simulink model "CF025A_GmFctDiArbn"  (R2013b)
settings: Solver=FixedStepDiscrete  SolverMode=SingleTasking  StartTime=0.0  StopTime=60  FixedStep=0.002  RelTol=1e-3
values from neighbouring files (symbols this model uses):
  GmFctDiArbnEotHwAgThd = DataDict.Calibration    [CF025A_GmFctDiArbn_DataDict.m]
  GmFctDiArbnEotTi = DataDict.Calibration    [CF025A_GmFctDiArbn_DataDict.m]
  GmFctDiArbnOnCentrHwAgThd = DataDict.Calibration    [CF025A_GmFctDiArbn_DataDict.m]
  GmFctDiArbnOnCentrHwTqThd = DataDict.Calibration    [CF025A_GmFctDiArbn_DataDict.m]
  GmFctDiArbnOnCentrTi = DataDict.Calibration    [CF025A_GmFctDiArbn_DataDict.m]
  GmFctDiArbnSrvTi = DataDict.Calibration    [CF025A_GmFctDiArbn_DataDict.m]
  MICROSECTOSEC_ULS_F32 = DataDict.Constant    [CF025A_GmFctDiArbn_DataDict.m]
  ZEROHWAG_HWDEG_F32 = DataDict.Constant    [CF025A_GmFctDiArbn_DataDict.m]
undefined symbols (not defined in the file or in its folder): GmFctDiArbnSts1, LoaSt1
libraries: simulink x7, FixdToFloat x4
(part 2 of 3)

== system CF025A_GmFctDiArbn/GmFctDiArbn/GmFctDiArbnPer1/LoaSt_doesnt_equal_SwBasdMtgtn/ComponentDisable/TimeOut ==
  Action Port : ActionPort  ActionType=then
  Constant{1..5} (5 alike) : Constant  Value=false
  Copyright1 : Subsystem  Description=|  mask(Copyright Information){none=on}
      | Copyright info block.                                               
      |                                                                     
      | Place copyright information at the top of every subsystem in design.
      mask prompts: none "No parameters"
      mask help: Place copyright information at the top of every subsystem in design.
      mask Display:
      | NxtrConf = 'Nexteer Confidential';
      | 
      | sys = bdroot; %handle for the current model ("system")
      | first = get_param(sys,'Created');
      | if(isempty(first))
      |     first = datestr(now,'yyyy');
      | else
      |     first = first(end-3:end);  %year is last four digits
      | end
      | 
      | last = get_param(sys,'LastModifiedDate');
      | if isempty(last)
      |     last = datestr(now,'yyyy');
      | else
      |     last = last(end-3:end);
      | end
      | 
      | if strcmp(first,last)
      |     fprintf('%s\nCopyright  %s Nexteer',NxtrConf,first);
      | else
      |     fprintf('%s\n%s%s-%s Nexteer',NxtrConf,char(169),first,last);
      | end
  Data Store Write : DataStoreWrite  DataStoreName=CcwEotEnad
  Data Store Write1 : DataStoreWrite  DataStoreName=CwEotEnad
  Enumerated Constant : simulink/Sources/Enumerated Constant  OutDataTypeStr=Enum: GmFctDiArbnSts1  Value=GmFctDiArbnSts1.GMFCTDIARBNSTS_TIMEOUTFAIL  SampleTime=inf
  WhlImbRejctnDi : Outport
  PullCmpActvDi : Outport  Port=2
  InertiaCmpDecelGainDi : Outport  Port=3
  GmFctDiSts_Out : Outport  Port=4
  wires:
  Enumerated Constant/1 -> GmFctDiSts_Out/1
  Constant3/1 -> InertiaCmpDecelGainDi/1
  Constant2/1 -> PullCmpActvDi/1
  Constant1/1 -> WhlImbRejctnDi/1
  Constant4/1 -> Data Store Write/1
  Constant5/1 -> Data Store Write1/1

== system CF025A_GmFctDiArbn/GmFctDiArbn/GmFctDiArbnPer1/LoaSt_doesnt_equal_SwBasdMtgtn/FcnDi_ElpdTi/Copyright1 ==

== system CF025A_GmFctDiArbn/GmFctDiArbn/GmFctDiArbnPer1/LoaSt_doesnt_equal_SwBasdMtgtn/FcnDi_ElpdTi/ElpdTi_TiPassd ==
  FcnDiStrtTi : Inport
  Action Port : ActionPort  ActionType=then
  Constant : Constant  Value=MICROSECTOSEC_ULS_F32
  Copyright1 : Subsystem  Description=|  mask(Copyright Information){none=on}
      | Copyright info block.                                               
      |                                                                     
      | Place copyright information at the top of every subsystem in design.
      mask prompts: none "No parameters"
      mask help: Place copyright information at the top of every subsystem in design.
      mask Display:
      | NxtrConf = 'Nexteer Confidential';
      | 
      | sys = bdroot; %handle for the current model ("system")
      | first = get_param(sys,'Created');
      | if(isempty(first))
      |     first = datestr(now,'yyyy');
      | else
      |     first = first(end-3:end);  %year is last four digits
      | end
      | 
      | last = get_param(sys,'LastModifiedDate');
      | if isempty(last)
      |     last = datestr(now,'yyyy');
      | else
      |     last = last(end-3:end);
      | end
      | 
      | if strcmp(first,last)
      |     fprintf('%s\nCopyright  %s Nexteer',NxtrConf,first);
      | else
      |     fprintf('%s\n%s%s-%s Nexteer',NxtrConf,char(169),first,last);
      | end
  FixdToFloat_f32_u32 : FixdToFloat/FixdToFloat_f32_u32  Param1=0
  GetTiSpan100MicroSec32bit : Subsystem
  Product : Product
  ElpdTi : Outport
  wires:
  GetTiSpan100MicroSec32bit/1(TiSpan) -> FixdToFloat_f32_u32/1
  FixdToFloat_f32_u32/1 -> Product/1
  Constant/1 -> Product/2
  FcnDiStrtTi/1 -> GetTiSpan100MicroSec32bit/1(RefTmr)
  Product/1 -> ElpdTi/1

== system CF025A_GmFctDiArbn/GmFctDiArbn/GmFctDiArbnPer1/LoaSt_doesnt_equal_SwBasdMtgtn/FcnDi_ElpdTi/ElpdTi_Zero ==
  Action Port : ActionPort  ActionType=else
  Constant : Constant  Value=0  OutDataTypeStr=single
  Copyright1 : Subsystem  Description=|  mask(Copyright Information){none=on}
      | Copyright info block.                                               
      |                                                                     
      | Place copyright information at the top of every subsystem in design.
      mask prompts: none "No parameters"
      mask help: Place copyright information at the top of every subsystem in design.
      mask Display:
      | NxtrConf = 'Nexteer Confidential';
      | 
      | sys = bdroot; %handle for the current model ("system")
      | first = get_param(sys,'Created');
      | if(isempty(first))
      |     first = datestr(now,'yyyy');
      | else
      |     first = first(end-3:end);  %year is last four digits
      | end
      | 
      | last = get_param(sys,'LastModifiedDate');
      | if isempty(last)
      |     last = datestr(now,'yyyy');
      | else
      |     last = last(end-3:end);
      | end
      | 
      | if strcmp(first,last)
      |     fprintf('%s\nCopyright  %s Nexteer',NxtrConf,first);
      | else
      |     fprintf('%s\n%s%s-%s Nexteer',NxtrConf,char(169),first,last);
      | end
  ElpdTi : Outport
  wires:
  Constant/1 -> ElpdTi/1

== system CF025A_GmFctDiArbn/GmFctDiArbn/GmFctDiArbnPer1/LoaSt_doesnt_equal_SwBasdMtgtn/CheckEotPosInRange/InProc/Copyright1 ==

== system CF025A_GmFctDiArbn/GmFctDiArbn/GmFctDiArbnPer1/LoaSt_doesnt_equal_SwBasdMtgtn/CheckEotPosInRange/InProc/InRangeCcwDirection ==
  CcwEot : Inport
  HwAgFinal : Inport  Port=2
  Action Port : ActionPort  ActionType=else
  Add : Sum
  Constant : Constant  Value=true
  Constant1 : Constant  Value=GmFctDiArbnEotTi
  Constant6 : Constant  Value=GmFctDiArbnEotHwAgThd
  Copyright1 : Subsystem  Description=|  mask(Copyright Information){none=on}
      | Copyright info block.                                               
      |                                                                     
      | Place copyright information at the top of every subsystem in design.
      mask prompts: none "No parameters"
      mask help: Place copyright information at the top of every subsystem in design.
      mask Display:
      | NxtrConf = 'Nexteer Confidential';
      | 
      | sys = bdroot; %handle for the current model ("system")
      | first = get_param(sys,'Created');
      | if(isempty(first))
      |     first = datestr(now,'yyyy');
      | else
      |     first = first(end-3:end);  %year is last four digits
      | end
      | 
      | last = get_param(sys,'LastModifiedDate');
      | if isempty(last)
      |     last = datestr(now,'yyyy');
      | else
      |     last = last(end-3:end);
      | end
      | 
      | if strcmp(first,last)
      |     fprintf('%s\nCopyright  %s Nexteer',NxtrConf,first);
      | else
      |     fprintf('%s\n%s%s-%s Nexteer',NxtrConf,char(169),first,last);
      | end
  Data Store Write : DataStoreWrite  DataStoreName=CcwEotEnad
  If : If  IfExpression=u1  ShowElse=off
  IfCcwElpdTiMet : Subsystem  TreatAsAtomicUnit=on
  InCcwEotElpdTi : Subsystem
  Relational Operator : RelationalOperator  OutDataTypeStr=boolean
  Relational Operator1 : RelationalOperator  OutDataTypeStr=boolean
  wires:
  CcwEot/1 -> Add/1
  Constant6/1 -> Add/2
  Constant/1 -> IfCcwElpdTiMet/1(In1)
  If/1 -> IfCcwElpdTiMet/Action
  IfCcwElpdTiMet/1(Out1) -> Data Store Write/1
  Add/1 -> Relational Operator/1
  HwAgFinal/1 -> Relational Operator/2
  InCcwEotElpdTi/1(ElpdTi) -> Relational Operator1/1
  Constant1/1 -> Relational Operator1/2
  Relational Operator1/1 -> If/1
  Relational Operator/1 -> InCcwEotElpdTi/1(InCcwEotRng)

== system CF025A_GmFctDiArbn/GmFctDiArbn/GmFctDiArbnPer1/LoaSt_doesnt_equal_SwBasdMtgtn/CheckEotPosInRange/InProc/InRangeCwDirection ==
  CwEot : Inport
  HwAgFinal : Inport  Port=2
  Action Port : ActionPort  ActionType=then
  Constant : Constant  Value=true
  Constant1 : Constant  Value=GmFctDiArbnEotTi
  Constant2 : Constant  Value=GmFctDiArbnEotHwAgThd
  Copyright1 : Subsystem  Description=|  mask(Copyright Information){none=on}
      | Copyright info block.                                               
      |                                                                     
      | Place copyright information at the top of every subsystem in design.
      mask prompts: none "No parameters"
      mask help: Place copyright information at the top of every subsystem in design.
      mask Display:
      | NxtrConf = 'Nexteer Confidential';
      | 
      | sys = bdroot; %handle for the current model ("system")
      | first = get_param(sys,'Created');
      | if(isempty(first))
      |     first = datestr(now,'yyyy');
      | else
      |     first = first(end-3:end);  %year is last four digits
      | end
      | 
      | last = get_param(sys,'LastModifiedDate');
      | if isempty(last)
      |     last = datestr(now,'yyyy');
      | else
      |     last = last(end-3:end);
      | end
      | 
      | if strcmp(first,last)
      |     fprintf('%s\nCopyright  %s Nexteer',NxtrConf,first);
      | else
      |     fprintf('%s\n%s%s-%s Nexteer',NxtrConf,char(169),first,last);
      | end
  Data Store Write : DataStoreWrite  DataStoreName=CwEotEnad
  If : If  IfExpression=u1  ShowElse=off
  IfCwEotElpdTiMet : Subsystem  TreatAsAtomicUnit=on
  InCwEotElpdTi : Subsystem
  Relational Operator : RelationalOperator  Operator=<=  OutDataTypeStr=boolean
  Relational Operator1 : RelationalOperator  OutDataTypeStr=boolean
  Subtract : Sum  Inputs=+-
  wires:
  CwEot/1 -> Subtract/1
  Constant2/1 -> Subtract/2
  Subtract/1 -> Relational Operator/1
  HwAgFinal/1 -> Relational Operator/2
  Relational Operator/1 -> InCwEotElpdTi/1(InCwEotRng)
  InCwEotElpdTi/1(ElpdTi) -> Relational Operator1/1
  Constant1/1 -> Relational Operator1/2
  Constant/1 -> IfCwEotElpdTiMet/1(In1)
  If/1 -> IfCwEotElpdTiMet/Action
  IfCwEotElpdTiMet/1(Out1) -> Data Store Write/1
  Relational Operator1/1 -> If/1

== system CF025A_GmFctDiArbn/GmFctDiArbn/GmFctDiArbnPer1/LoaSt_doesnt_equal_SwBasdMtgtn/CheckEotPosInRange/Wait/Copyright1 ==

== system CF025A_GmFctDiArbn/GmFctDiArbn/GmFctDiArbnPer1/LoaSt_doesnt_equal_SwBasdMtgtn/CheckHwTqZeroAndHwAgZero/IfBothEotElpdTimeMet/Copyright1 ==

== system CF025A_GmFctDiArbn/GmFctDiArbn/GmFctDiArbnPer1/LoaSt_doesnt_equal_SwBasdMtgtn/CheckHwTqZeroAndHwAgZero/IfBothEotElpdTimeMet/OnCentrElpdTi ==
  InOnCentrRng : Inport
  Copyright1 : Subsystem  Description=|  mask(Copyright Information){none=on}
      | Copyright info block.                                               
      |                                                                     
      | Place copyright information at the top of every subsystem in design.
      mask prompts: none "No parameters"
      mask help: Place copyright information at the top of every subsystem in design.
      mask Display:
      | NxtrConf = 'Nexteer Confidential';
      | 
      | sys = bdroot; %handle for the current model ("system")
      | first = get_param(sys,'Created');
      | if(isempty(first))
      |     first = datestr(now,'yyyy');
      | else
      |     first = first(end-3:end);  %year is last four digits
      | end
      | 
      | last = get_param(sys,'LastModifiedDate');
      | if isempty(last)
      |     last = datestr(now,'yyyy');
      | else
      |     last = last(end-3:end);
      | end
      | 
      | if strcmp(first,last)
      |     fprintf('%s\nCopyright  %s Nexteer',NxtrConf,first);
      | else
      |     fprintf('%s\n%s%s-%s Nexteer',NxtrConf,char(169),first,last);
      | end
  Data Store Read : DataStoreRead  DataStoreName=InOnCentrRng
  ElpdTi_Check : Subsystem  TreatAsAtomicUnit=on
  ElpdTi_Start : Subsystem  TreatAsAtomicUnit=on
  ElpdTi_Zero : Subsystem  TreatAsAtomicUnit=on
  If : If  NumInputs=2  IfExpression=u1  ElseIfExpressions=u2
  Logical Operator : Logic  Operator=NOT  AllPortsSameDT=off  OutDataTypeStr=boolean
  Logical Operator1 : Logic  Operator=NOT  AllPortsSameDT=off  OutDataTypeStr=boolean
  Merge : Merge  Inputs=3
  ElpdTi : Outport
  wires:
  If/1 -> ElpdTi_Zero/Action
  If/3 -> ElpdTi_Check/Action
  InOnCentrRng/1 -> Logical Operator1/1
  Logical Operator1/1 -> If/1
  Data Store Read/1 -> Logical Operator/1
  Merge/1 -> ElpdTi/1
  Logical Operator/1 -> If/2
  ElpdTi_Check/1(ElpdTi) -> Merge/3
  ElpdTi_Start/1(ElpdTi) -> Merge/2
  If/2 -> ElpdTi_Start/Action
  ElpdTi_Zero/1(ElpdTi) -> Merge/1

== system CF025A_GmFctDiArbn/GmFctDiArbn/GmFctDiArbnPer1/LoaSt_doesnt_equal_SwBasdMtgtn/ComponentDisable/Disabled/Copyright1 ==

== system CF025A_GmFctDiArbn/GmFctDiArbn/GmFctDiArbnPer1/LoaSt_doesnt_equal_SwBasdMtgtn/ComponentDisable/NoDisable/Copyright1 ==

== system CF025A_GmFctDiArbn/GmFctDiArbn/GmFctDiArbnPer1/LoaSt_doesnt_equal_SwBasdMtgtn/ComponentDisable/TimeOut/Copyright1 ==

== system CF025A_GmFctDiArbn/GmFctDiArbn/GmFctDiArbnPer1/LoaSt_doesnt_equal_SwBasdMtgtn/FcnDi_ElpdTi/ElpdTi_TiPassd/Copyright1 ==

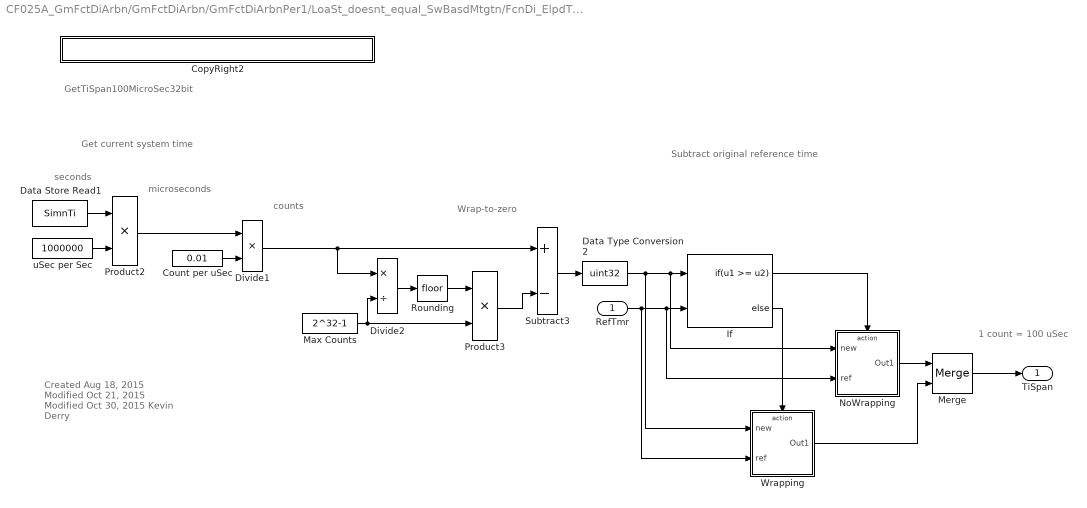
== system CF025A_GmFctDiArbn/GmFctDiArbn/GmFctDiArbnPer1/LoaSt_doesnt_equal_SwBasdMtgtn/FcnDi_ElpdTi/ElpdTi_TiPassd/GetTiSpan100MicroSec32bit ==
  note: Created Aug 18, 2015
      | Modified Oct 21, 2015
      | Modified Oct 30, 2015
      | Kevin Derry
  note: GetTiSpan100MicroSec32bit
  note: Get current system time
  note: 1 count = 100 uSec
  note: Wrap-to-zero
  note: counts
  note: microseconds
  note: seconds
  note: Subtract original reference time
  RefTmr : Inport
  CopyRight2 : Subsystem  Description=|  mask(Copyright Information){none=on}
      | Copyright info block.                                               
      |                                                                     
      | Place copyright information at the top of every subsystem in design.
      mask prompts: none "No parameters"
      mask help: Place copyright information at the top of every subsystem in design.
      mask Display:
      | NxtrConf = 'Nexteer Confidential';
      | 
      | sys = bdroot; %handle for the current model ("system")
      | first = get_param(sys,'Created');
      | if(isempty(first))
      |     first = datestr(now,'yyyy');
      | else
      |     first = first(end-3:end);  %year is last four digits
      | end
      | 
      | last = get_param(sys,'LastModifiedDate');
      | if isempty(last)
      |     last = datestr(now,'yyyy');
      | else
      |     last = last(end-3:end);
      | end
      | 
      | if strcmp(first,last)
      |     fprintf('%s -- Copyright %s Nexteer',NxtrConf,first)
      | else
      |     fprintf('%s -- %s%s- %s Nexteer',NxtrConf,char(169),first,last)
      | end
  Count per uSec : Constant  Value=0.01
  Data Store Read1 : DataStoreRead  DataStoreName=SimnTi
  Data Type Conversion2 : DataTypeConversion  OutDataTypeStr=uint32
  Divide1 : Product  Inputs=**
  Divide2 : Product  Inputs=*/
  If : If  NumInputs=2  IfExpression=u1 >= u2
  Max Counts : Constant  Value=2^32-1
  Merge : Merge
  NoWrapping : Subsystem  TreatAsAtomicUnit=on
  Product2 : Product
  Product3 : Product
  Rounding : Rounding
  Subtract3 : Sum  Inputs=+-
  Wrapping : Subsystem  TreatAsAtomicUnit=on
  uSec per Sec : Constant  Value=1000000
  TiSpan : Outport
  wires:
  Data Type Conversion2/1 -> Wrapping/1(new), NoWrapping/1(new), If/1
  RefTmr/1 -> Wrapping/2(ref), NoWrapping/2(ref), If/2
  Merge/1 -> TiSpan/1
  uSec per Sec/1 -> Product2/2
  Count per uSec/1 -> Divide1/2
  Data Store Read1/1 -> Product2/1
  Product2/1 -> Divide1/1
  Divide1/1 -> Subtract3/1, Divide2/1
  Max Counts/1 -> Product3/2, Divide2/2
  Divide2/1 -> Rounding/1
  Rounding/1 -> Product3/1
  Subtract3/1 -> Data Type Conversion2/1
  Product3/1 -> Subtract3/2
  If/1 -> NoWrapping/Action
  If/2 -> Wrapping/Action
  NoWrapping/1(Out1) -> Merge/1
  Wrapping/1(Out1) -> Merge/2

== system CF025A_GmFctDiArbn/GmFctDiArbn/GmFctDiArbnPer1/LoaSt_doesnt_equal_SwBasdMtgtn/FcnDi_ElpdTi/ElpdTi_Zero/Copyright1 ==

== system CF025A_GmFctDiArbn/GmFctDiArbn/GmFctDiArbnPer1/LoaSt_doesnt_equal_SwBasdMtgtn/CheckEotPosInRange/InProc/InRangeCcwDirection/Copyright1 ==

== system CF025A_GmFctDiArbn/GmFctDiArbn/GmFctDiArbnPer1/LoaSt_doesnt_equal_SwBasdMtgtn/CheckEotPosInRange/InProc/InRangeCcwDirection/IfCcwElpdTiMet ==
  In1 : Inport
  Action Port : ActionPort  ActionType=then
  Out1 : Outport
  wires:
  In1/1 -> Out1/1

== system CF025A_GmFctDiArbn/GmFctDiArbn/GmFctDiArbnPer1/LoaSt_doesnt_equal_SwBasdMtgtn/CheckEotPosInRange/InProc/InRangeCcwDirection/InCcwEotElpdTi ==
  InCcwEotRng : Inport
  Data Store Read : DataStoreRead  DataStoreName=InCcwEotRng
  ElpdTi_Check : Subsystem  TreatAsAtomicUnit=on
  ElpdTi_Start : Subsystem  TreatAsAtomicUnit=on
  ElpdTi_Zero : Subsystem  TreatAsAtomicUnit=on
  If : If  NumInputs=2  IfExpression=u1  ElseIfExpressions=u2
  Logical Operator : Logic  Operator=NOT  AllPortsSameDT=off  OutDataTypeStr=boolean
  Logical Operator1 : Logic  Operator=NOT  AllPortsSameDT=off  OutDataTypeStr=boolean
  Merge : Merge  Inputs=3
  ElpdTi : Outport
  wires:
  ElpdTi_Zero/1(ElpdTi) -> Merge/3
  ElpdTi_Start/1(ElpdTi) -> Merge/2
  ElpdTi_Check/1(ElpdTi) -> Merge/1
  If/2 -> ElpdTi_Start/Action
  Logical Operator/1 -> If/2
  Merge/1 -> ElpdTi/1
  Data Store Read/1 -> Logical Operator/1
  Logical Operator1/1 -> If/1
  InCcwEotRng/1 -> Logical Operator1/1
  If/3 -> ElpdTi_Check/Action
  If/1 -> ElpdTi_Zero/Action

== system CF025A_GmFctDiArbn/GmFctDiArbn/GmFctDiArbnPer1/LoaSt_doesnt_equal_SwBasdMtgtn/CheckEotPosInRange/InProc/InRangeCwDirection/Copyright1 ==

== system CF025A_GmFctDiArbn/GmFctDiArbn/GmFctDiArbnPer1/LoaSt_doesnt_equal_SwBasdMtgtn/CheckEotPosInRange/InProc/InRangeCwDirection/IfCwEotElpdTiMet ==
  In1 : Inport
  Action Port : ActionPort  ActionType=then
  Copyright1 : Subsystem  Description=|  mask(Copyright Information){none=on}
      | Copyright info block.                                               
      |                                                                     
      | Place copyright information at the top of every subsystem in design.
      mask prompts: none "No parameters"
      mask help: Place copyright information at the top of every subsystem in design.
      mask Display:
      | NxtrConf = 'Nexteer Confidential';
      | 
      | sys = bdroot; %handle for the current model ("system")
      | first = get_param(sys,'Created');
      | if(isempty(first))
      |     first = datestr(now,'yyyy');
      | else
      |     first = first(end-3:end);  %year is last four digits
      | end
      | 
      | last = get_param(sys,'LastModifiedDate');
      | if isempty(last)
      |     last = datestr(now,'yyyy');
      | else
      |     last = last(end-3:end);
      | end
      | 
      | if strcmp(first,last)
      |     fprintf('%s\nCopyright  %s Nexteer',NxtrConf,first);
      | else
      |     fprintf('%s\n%s%s-%s Nexteer',NxtrConf,char(169),first,last);
      | end
  Out1 : Outport
  wires:
  In1/1 -> Out1/1

== system CF025A_GmFctDiArbn/GmFctDiArbn/GmFctDiArbnPer1/LoaSt_doesnt_equal_SwBasdMtgtn/CheckEotPosInRange/InProc/InRangeCwDirection/InCwEotElpdTi ==
  InCwEotRng : Inport
  Copyright1 : Subsystem  Description=|  mask(Copyright Information){none=on}
      | Copyright info block.                                               
      |                                                                     
      | Place copyright information at the top of every subsystem in design.
      mask prompts: none "No parameters"
      mask help: Place copyright information at the top of every subsystem in design.
      mask Display:
      | NxtrConf = 'Nexteer Confidential';
      | 
      | sys = bdroot; %handle for the current model ("system")
      | first = get_param(sys,'Created');
      | if(isempty(first))
      |     first = datestr(now,'yyyy');
      | else
      |     first = first(end-3:end);  %year is last four digits
      | end
      | 
      | last = get_param(sys,'LastModifiedDate');
      | if isempty(last)
      |     last = datestr(now,'yyyy');
      | else
      |     last = last(end-3:end);
      | end
      | 
      | if strcmp(first,last)
      |     fprintf('%s\nCopyright  %s Nexteer',NxtrConf,first);
      | else
      |     fprintf('%s\n%s%s-%s Nexteer',NxtrConf,char(169),first,last);
      | end
  Data Store Read : DataStoreRead  DataStoreName=InCwEotRng
  ElpdTi_Check : Subsystem  TreatAsAtomicUnit=on
  ElpdTi_Start : Subsystem  TreatAsAtomicUnit=on
  ElpdTi_Zero : Subsystem  TreatAsAtomicUnit=on
  If : If  NumInputs=2  IfExpression=u1  ElseIfExpressions=u2
  Logical Operator : Logic  Operator=NOT  AllPortsSameDT=off  OutDataTypeStr=boolean
  Logical Operator1 : Logic  Operator=NOT  AllPortsSameDT=off  OutDataTypeStr=boolean
  Merge : Merge  Inputs=3
  ElpdTi : Outport
  wires:
  If/1 -> ElpdTi_Zero/Action
  If/3 -> ElpdTi_Check/Action
  InCwEotRng/1 -> Logical Operator1/1
  Logical Operator1/1 -> If/1
  Data Store Read/1 -> Logical Operator/1
  Merge/1 -> ElpdTi/1
  Logical Operator/1 -> If/2
  If/2 -> ElpdTi_Start/Action
  ElpdTi_Check/1(ElpdTi) -> Merge/1
  ElpdTi_Start/1(ElpdTi) -> Merge/2
  ElpdTi_Zero/1(ElpdTi) -> Merge/3

== system CF025A_GmFctDiArbn/GmFctDiArbn/GmFctDiArbnPer1/LoaSt_doesnt_equal_SwBasdMtgtn/CheckHwTqZeroAndHwAgZero/IfBothEotElpdTimeMet/OnCentrElpdTi/Copyright1 ==

== system CF025A_GmFctDiArbn/GmFctDiArbn/GmFctDiArbnPer1/LoaSt_doesnt_equal_SwBasdMtgtn/CheckHwTqZeroAndHwAgZero/IfBothEotElpdTimeMet/OnCentrElpdTi/ElpdTi_Check ==
  Action Port : ActionPort  ActionType=else
  Constant : Constant  Value=MICROSECTOSEC_ULS_F32
  Constant1 : Constant  Value=true
  Copyright1 : Subsystem  Description=|  mask(Copyright Information){none=on}
      | Copyright info block.                                               
      |                                                                     
      | Place copyright information at the top of every subsystem in design.
      mask prompts: none "No parameters"
      mask help: Place copyright information at the top of every subsystem in design.
      mask Display:
      | NxtrConf = 'Nexteer Confidential';
      | 
      | sys = bdroot; %handle for the current model ("system")
      | first = get_param(sys,'Created');
      | if(isempty(first))
      |     first = datestr(now,'yyyy');
      | else
      |     first = first(end-3:end);  %year is last four digits
      | end
      | 
      | last = get_param(sys,'LastModifiedDate');
      | if isempty(last)
      |     last = datestr(now,'yyyy');
      | else
      |     last = last(end-3:end);
      | end
      | 
      | if strcmp(first,last)
      |     fprintf('%s\nCopyright  %s Nexteer',NxtrConf,first);
      | else
      |     fprintf('%s\n%s%s-%s Nexteer',NxtrConf,char(169),first,last);
      | end
  Data Store Read : DataStoreRead  DataStoreName=OnCentrElpdTi
  Data Store Write1 : DataStoreWrite  DataStoreName=InOnCentrRng
  FixdToFloat_f32_u32 : FixdToFloat/FixdToFloat_f32_u32  Param1=0
  GetTiSpan100MicroSec32bit : Subsystem
  Product : Product
  ElpdTi : Outport
  wires:
  Constant1/1 -> Data Store Write1/1
  Data Store Read/1 -> GetTiSpan100MicroSec32bit/1(RefTmr)
  GetTiSpan100MicroSec32bit/1(TiSpan) -> FixdToFloat_f32_u32/1
  FixdToFloat_f32_u32/1 -> Product/1
  Product/1 -> ElpdTi/1
  Constant/1 -> Product/2

== system CF025A_GmFctDiArbn/GmFctDiArbn/GmFctDiArbnPer1/LoaSt_doesnt_equal_SwBasdMtgtn/CheckHwTqZeroAndHwAgZero/IfBothEotElpdTimeMet/OnCentrElpdTi/ElpdTi_Start ==
  Action Port : ActionPort  ActionType=elseif
  Constant : Constant  Value=0  OutDataTypeStr=single
  Constant1 : Constant  Value=true
  Copyright1 : Subsystem  Description=|  mask(Copyright Information){none=on}
      | Copyright info block.                                               
      |                                                                     
      | Place copyright information at the top of every subsystem in design.
      mask prompts: none "No parameters"
      mask help: Place copyright information at the top of every subsystem in design.
      mask Display:
      | NxtrConf = 'Nexteer Confidential';
      | 
      | sys = bdroot; %handle for the current model ("system")
      | first = get_param(sys,'Created');
      | if(isempty(first))
      |     first = datestr(now,'yyyy');
      | else
      |     first = first(end-3:end);  %year is last four digits
      | end
      | 
      | last = get_param(sys,'LastModifiedDate');
      | if isempty(last)
      |     last = datestr(now,'yyyy');
      | else
      |     last = last(end-3:end);
      | end
      | 
      | if strcmp(first,last)
      |     fprintf('%s\nCopyright  %s Nexteer',NxtrConf,first);
      | else
      |     fprintf('%s\n%s%s-%s Nexteer',NxtrConf,char(169),first,last);
      | end
  Data Store Write : DataStoreWrite  DataStoreName=OnCentrElpdTi
  Data Store Write1 : DataStoreWrite  DataStoreName=InOnCentrRng
  GetRefTmr100MicroSec32bit : Subsystem
  ElpdTi : Outport
  wires:
  GetRefTmr100MicroSec32bit/1(RefTmr) -> Data Store Write/1
  Constant/1 -> ElpdTi/1
  Constant1/1 -> Data Store Write1/1

== system CF025A_GmFctDiArbn/GmFctDiArbn/GmFctDiArbnPer1/LoaSt_doesnt_equal_SwBasdMtgtn/CheckHwTqZeroAndHwAgZero/IfBothEotElpdTimeMet/OnCentrElpdTi/ElpdTi_Zero ==
  Action Port : ActionPort  ActionType=then
  Constant1 : Constant  Value=0  OutDataTypeStr=single
  Constant2 : Constant  Value=false
  Copyright1 : Subsystem  Description=|  mask(Copyright Information){none=on}
      | Copyright info block.                                               
      |                                                                     
      | Place copyright information at the top of every subsystem in design.
      mask prompts: none "No parameters"
      mask help: Place copyright information at the top of every subsystem in design.
      mask Display:
      | NxtrConf = 'Nexteer Confidential';
      | 
      | sys = bdroot; %handle for the current model ("system")
      | first = get_param(sys,'Created');
      | if(isempty(first))
      |     first = datestr(now,'yyyy');
      | else
      |     first = first(end-3:end);  %year is last four digits
      | end
      | 
      | last = get_param(sys,'LastModifiedDate');
      | if isempty(last)
      |     last = datestr(now,'yyyy');
      | else
      |     last = last(end-3:end);
      | end
      | 
      | if strcmp(first,last)
      |     fprintf('%s\nCopyright  %s Nexteer',NxtrConf,first);
      | else
      |     fprintf('%s\n%s%s-%s Nexteer',NxtrConf,char(169),first,last);
      | end
  Data Store Write2 : DataStoreWrite  DataStoreName=InOnCentrRng
  ElpdTi : Outport
  wires:
  Constant1/1 -> ElpdTi/1
  Constant2/1 -> Data Store Write2/1

== system CF025A_GmFctDiArbn/GmFctDiArbn/GmFctDiArbnPer1/LoaSt_doesnt_equal_SwBasdMtgtn/FcnDi_ElpdTi/ElpdTi_TiPassd/GetTiSpan100MicroSec32bit/CopyRight2 ==

== system CF025A_GmFctDiArbn/GmFctDiArbn/GmFctDiArbnPer1/LoaSt_doesnt_equal_SwBasdMtgtn/FcnDi_ElpdTi/ElpdTi_TiPassd/GetTiSpan100MicroSec32bit/NoWrapping ==
  new : Inport
  ref : Inport  Port=2
  Action Port : ActionPort  ActionType=then
  CopyRight2 : Subsystem  Description=|  mask(Copyright Information){none=on}
      | Copyright info block.                                               
      |                                                                     
      | Place copyright information at the top of every subsystem in design.
      mask prompts: none "No parameters"
      mask help: Place copyright information at the top of every subsystem in design.
      mask Display:
      | NxtrConf = 'Nexteer Confidential';
      | 
      | sys = bdroot; %handle for the current model ("system")
      | first = get_param(sys,'Created');
      | if(isempty(first))
      |     first = datestr(now,'yyyy');
      | else
      |     first = first(end-3:end);  %year is last four digits
      | end
      | 
      | last = get_param(sys,'LastModifiedDate');
      | if isempty(last)
      |     last = datestr(now,'yyyy');
      | else
      |     last = last(end-3:end);
      | end
      | 
      | if strcmp(first,last)
      |     fprintf('%s -- Copyright %s Nexteer',NxtrConf,first)
      | else
      |     fprintf('%s -- %s%s- %s Nexteer',NxtrConf,char(169),first,last)
      | end
  Subtract1 : Sum  Inputs=+-
  Out1 : Outport
  wires:
  Subtract1/1 -> Out1/1
  new/1 -> Subtract1/1
  ref/1 -> Subtract1/2

== system CF025A_GmFctDiArbn/GmFctDiArbn/GmFctDiArbnPer1/LoaSt_doesnt_equal_SwBasdMtgtn/FcnDi_ElpdTi/ElpdTi_TiPassd/GetTiSpan100MicroSec32bit/Wrapping ==
  new : Inport
  ref : Inport  Port=2
  Action Port : ActionPort  ActionType=else
  CopyRight2 : Subsystem  Description=|  mask(Copyright Information){none=on}
      | Copyright info block.                                               
      |                                                                     
      | Place copyright information at the top of every subsystem in design.
      mask prompts: none "No parameters"
      mask help: Place copyright information at the top of every subsystem in design.
      mask Display:
      | NxtrConf = 'Nexteer Confidential';
      | 
      | sys = bdroot; %handle for the current model ("system")
      | first = get_param(sys,'Created');
      | if(isempty(first))
      |     first = datestr(now,'yyyy');
      | else
      |     first = first(end-3:end);  %year is last four digits
      | end
      | 
      | last = get_param(sys,'LastModifiedDate');
      | if isempty(last)
      |     last = datestr(now,'yyyy');
      | else
      |     last = last(end-3:end);
      | end
      | 
      | if strcmp(first,last)
      |     fprintf('%s -- Copyright %s Nexteer',NxtrConf,first)
      | else
      |     fprintf('%s -- %s%s- %s Nexteer',NxtrConf,char(169),first,last)
      | end
  Max Counts : Constant  Value=2^32-1  OutDataTypeStr=uint32
  Subtract1 : Sum  Inputs=+-+
  Out1 : Outport
  wires:
  Subtract1/1 -> Out1/1
  Max Counts/1 -> Subtract1/1
  ref/1 -> Subtract1/2
  new/1 -> Subtract1/3

== system CF025A_GmFctDiArbn/GmFctDiArbn/GmFctDiArbnPer1/LoaSt_doesnt_equal_SwBasdMtgtn/CheckEotPosInRange/InProc/InRangeCcwDirection/InCcwEotElpdTi/ElpdTi_Check ==
  Action Port : ActionPort  ActionType=else
  Constant : Constant  Value=MICROSECTOSEC_ULS_F32
  Constant1 : Constant  Value=true
  Data Store Read : DataStoreRead  DataStoreName=InCcwEotRngElpdTi
  Data Store Write2 : DataStoreWrite  DataStoreName=InCcwEotRng
  FixdToFloat_f32_u32 : FixdToFloat/FixdToFloat_f32_u32  Param1=0
  GetTiSpan100MicroSec32bit : Subsystem
  Product : Product
  ElpdTi : Outport
  wires:
  Constant/1 -> Product/2
  Product/1 -> ElpdTi/1
  FixdToFloat_f32_u32/1 -> Product/1
  GetTiSpan100MicroSec32bit/1(TiSpan) -> FixdToFloat_f32_u32/1
  Data Store Read/1 -> GetTiSpan100MicroSec32bit/1(RefTmr)
  Constant1/1 -> Data Store Write2/1

== system CF025A_GmFctDiArbn/GmFctDiArbn/GmFctDiArbnPer1/LoaSt_doesnt_equal_SwBasdMtgtn/CheckEotPosInRange/InProc/InRangeCcwDirection/InCcwEotElpdTi/ElpdTi_Start ==
  Action Port : ActionPort  ActionType=elseif
  Constant : Constant  Value=0  OutDataTypeStr=single
  Constant1 : Constant  Value=true
  Data Store Write : DataStoreWrite  DataStoreName=InCcwEotRngElpdTi
  Data Store Write2 : DataStoreWrite  DataStoreName=InCcwEotRng
  GetRefTmr100MicroSec32bit : Subsystem
  ElpdTi : Outport
  wires:
  Constant1/1 -> Data Store Write2/1
  Constant/1 -> ElpdTi/1
  GetRefTmr100MicroSec32bit/1(RefTmr) -> Data Store Write/1

== system CF025A_GmFctDiArbn/GmFctDiArbn/GmFctDiArbnPer1/LoaSt_doesnt_equal_SwBasdMtgtn/CheckEotPosInRange/InProc/InRangeCcwDirection/InCcwEotElpdTi/ElpdTi_Zero ==
  Action Port : ActionPort  ActionType=then
  Constant1 : Constant  Value=0  OutDataTypeStr=single
  Constant2 : Constant  Value=false
  Data Store Write2 : DataStoreWrite  DataStoreName=InCcwEotRng
  ElpdTi : Outport
  wires:
  Constant2/1 -> Data Store Write2/1
  Constant1/1 -> ElpdTi/1

== system CF025A_GmFctDiArbn/GmFctDiArbn/GmFctDiArbnPer1/LoaSt_doesnt_equal_SwBasdMtgtn/CheckEotPosInRange/InProc/InRangeCwDirection/IfCwEotElpdTiMet/Copyright1 ==

== system CF025A_GmFctDiArbn/GmFctDiArbn/GmFctDiArbnPer1/LoaSt_doesnt_equal_SwBasdMtgtn/CheckEotPosInRange/InProc/InRangeCwDirection/InCwEotElpdTi/Copyright1 ==

== system CF025A_GmFctDiArbn/GmFctDiArbn/GmFctDiArbnPer1/LoaSt_doesnt_equal_SwBasdMtgtn/CheckEotPosInRange/InProc/InRangeCwDirection/InCwEotElpdTi/ElpdTi_Check ==
  Action Port : ActionPort  ActionType=else
  Constant : Constant  Value=MICROSECTOSEC_ULS_F32
  Constant1 : Constant  Value=true
  Copyright1 : Subsystem  Description=|  mask(Copyright Information){none=on}
      | Copyright info block.                                               
      |                                                                     
      | Place copyright information at the top of every subsystem in design.
      mask prompts: none "No parameters"
      mask help: Place copyright information at the top of every subsystem in design.
      mask Display:
      | NxtrConf = 'Nexteer Confidential';
      | 
      | sys = bdroot; %handle for the current model ("system")
      | first = get_param(sys,'Created');
      | if(isempty(first))
      |     first = datestr(now,'yyyy');
      | else
      |     first = first(end-3:end);  %year is last four digits
      | end
      | 
      | last = get_param(sys,'LastModifiedDate');
      | if isempty(last)
      |     last = datestr(now,'yyyy');
      | else
      |     last = last(end-3:end);
      | end
      | 
      | if strcmp(first,last)
      |     fprintf('%s\nCopyright  %s Nexteer',NxtrConf,first);
      | else
      |     fprintf('%s\n%s%s-%s Nexteer',NxtrConf,char(169),first,last);
      | end
  Data Store Read : DataStoreRead  DataStoreName=InCwEotRngElpdTi
  Data Store Write2 : DataStoreWrite  DataStoreName=InCwEotRng
  FixdToFloat_f32_u32 : FixdToFloat/FixdToFloat_f32_u32  Param1=0
  GetTiSpan100MicroSec32bit : Subsystem
  Product : Product
  ElpdTi : Outport
  wires:
  Constant1/1 -> Data Store Write2/1
  Data Store Read/1 -> GetTiSpan100MicroSec32bit/1(RefTmr)
  GetTiSpan100MicroSec32bit/1(TiSpan) -> FixdToFloat_f32_u32/1
  FixdToFloat_f32_u32/1 -> Product/1
  Product/1 -> ElpdTi/1
  Constant/1 -> Product/2

== system CF025A_GmFctDiArbn/GmFctDiArbn/GmFctDiArbnPer1/LoaSt_doesnt_equal_SwBasdMtgtn/CheckEotPosInRange/InProc/InRangeCwDirection/InCwEotElpdTi/ElpdTi_Start ==
  Action Port : ActionPort  ActionType=elseif
  Constant : Constant  Value=0  OutDataTypeStr=single
  Constant1 : Constant  Value=true
  Copyright1 : Subsystem  Description=|  mask(Copyright Information){none=on}
      | Copyright info block.                                               
      |                                                                     
      | Place copyright information at the top of every subsystem in design.
      mask prompts: none "No parameters"
      mask help: Place copyright information at the top of every subsystem in design.
      mask Display:
      | NxtrConf = 'Nexteer Confidential';
      | 
      | sys = bdroot; %handle for the current model ("system")
      | first = get_param(sys,'Created');
      | if(isempty(first))
      |     first = datestr(now,'yyyy');
      | else
      |     first = first(end-3:end);  %year is last four digits
      | end
      | 
      | last = get_param(sys,'LastModifiedDate');
      | if isempty(last)
      |     last = datestr(now,'yyyy');
      | else
      |     last = last(end-3:end);
      | end
      | 
      | if strcmp(first,last)
      |     fprintf('%s\nCopyright  %s Nexteer',NxtrConf,first);
      | else
      |     fprintf('%s\n%s%s-%s Nexteer',NxtrConf,char(169),first,last);
      | end
  Data Store Write : DataStoreWrite  DataStoreName=InCwEotRngElpdTi
  Data Store Write2 : DataStoreWrite  DataStoreName=InCwEotRng
  GetRefTmr100MicroSec32bit : Subsystem
  ElpdTi : Outport
  wires:
  GetRefTmr100MicroSec32bit/1(RefTmr) -> Data Store Write/1
  Constant/1 -> ElpdTi/1
  Constant1/1 -> Data Store Write2/1

== system CF025A_GmFctDiArbn/GmFctDiArbn/GmFctDiArbnPer1/LoaSt_doesnt_equal_SwBasdMtgtn/CheckEotPosInRange/InProc/InRangeCwDirection/InCwEotElpdTi/ElpdTi_Zero ==
  Action Port : ActionPort  ActionType=then
  Constant1 : Constant  Value=0  OutDataTypeStr=single
  Constant2 : Constant  Value=false
  Copyright1 : Subsystem  Description=|  mask(Copyright Information){none=on}
      | Copyright info block.                                               
      |                                                                     
      | Place copyright information at the top of every subsystem in design.
      mask prompts: none "No parameters"
      mask help: Place copyright information at the top of every subsystem in design.
      mask Display:
      | NxtrConf = 'Nexteer Confidential';
      | 
      | sys = bdroot; %handle for the current model ("system")
      | first = get_param(sys,'Created');
      | if(isempty(first))
      |     first = datestr(now,'yyyy');
      | else
      |     first = first(end-3:end);  %year is last four digits
      | end
      | 
      | last = get_param(sys,'LastModifiedDate');
      | if isempty(last)
      |     last = datestr(now,'yyyy');
      | else
      |     last = last(end-3:end);
      | end
      | 
      | if strcmp(first,last)
      |     fprintf('%s\nCopyright  %s Nexteer',NxtrConf,first);
      | else
      |     fprintf('%s\n%s%s-%s Nexteer',NxtrConf,char(169),first,last);
      | end
  Data Store Write2 : DataStoreWrite  DataStoreName=InCwEotRng
  ElpdTi : Outport
  wires:
  Constant1/1 -> ElpdTi/1
  Constant2/1 -> Data Store Write2/1

== system CF025A_GmFctDiArbn/GmFctDiArbn/GmFctDiArbnPer1/LoaSt_doesnt_equal_SwBasdMtgtn/CheckHwTqZeroAndHwAgZero/IfBothEotElpdTimeMet/OnCentrElpdTi/ElpdTi_Check/Copyright1 ==

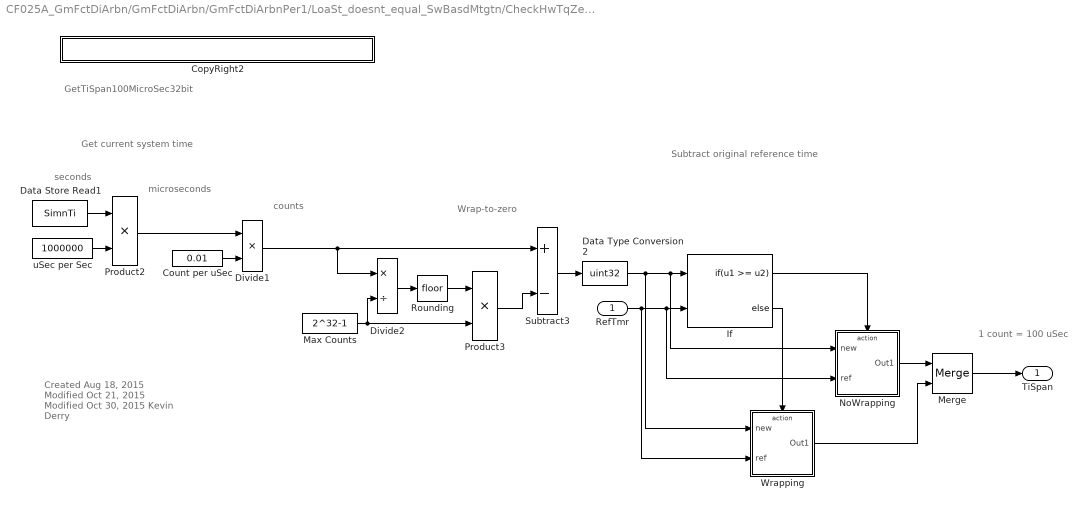
== system CF025A_GmFctDiArbn/GmFctDiArbn/GmFctDiArbnPer1/LoaSt_doesnt_equal_SwBasdMtgtn/CheckHwTqZeroAndHwAgZero/IfBothEotElpdTimeMet/OnCentrElpdTi/ElpdTi_Check/GetTiSpan100MicroSec32bit ==
  note: Created Aug 18, 2015
      | Modified Oct 21, 2015
      | Modified Oct 30, 2015
      | Kevin Derry
  note: GetTiSpan100MicroSec32bit
  note: Get current system time
  note: 1 count = 100 uSec
  note: Wrap-to-zero
  note: counts
  note: microseconds
  note: seconds
  note: Subtract original reference time
  RefTmr : Inport
  CopyRight2 : Subsystem  Description=|  mask(Copyright Information){none=on}
      | Copyright info block.                                               
      |                                                                     
      | Place copyright information at the top of every subsystem in design.
      mask prompts: none "No parameters"
      mask help: Place copyright information at the top of every subsystem in design.
      mask Display:
      | NxtrConf = 'Nexteer Confidential';
      | 
      | sys = bdroot; %handle for the current model ("system")
      | first = get_param(sys,'Created');
      | if(isempty(first))
      |     first = datestr(now,'yyyy');
      | else
      |     first = first(end-3:end);  %year is last four digits
      | end
      | 
      | last = get_param(sys,'LastModifiedDate');
      | if isempty(last)
      |     last = datestr(now,'yyyy');
      | else
      |     last = last(end-3:end);
      | end
      | 
      | if strcmp(first,last)
      |     fprintf('%s -- Copyright %s Nexteer',NxtrConf,first)
      | else
      |     fprintf('%s -- %s%s- %s Nexteer',NxtrConf,char(169),first,last)
      | end
  Count per uSec : Constant  Value=0.01
  Data Store Read1 : DataStoreRead  DataStoreName=SimnTi
  Data Type Conversion2 : DataTypeConversion  OutDataTypeStr=uint32
  Divide1 : Product  Inputs=**
  Divide2 : Product  Inputs=*/
  If : If  NumInputs=2  IfExpression=u1 >= u2
  Max Counts : Constant  Value=2^32-1
  Merge : Merge
  NoWrapping : Subsystem  TreatAsAtomicUnit=on
  Product2 : Product
  Product3 : Product
  Rounding : Rounding
  Subtract3 : Sum  Inputs=+-
  Wrapping : Subsystem  TreatAsAtomicUnit=on
  uSec per Sec : Constant  Value=1000000
  TiSpan : Outport
  wires:
  Data Type Conversion2/1 -> Wrapping/1(new), NoWrapping/1(new), If/1
  RefTmr/1 -> Wrapping/2(ref), NoWrapping/2(ref), If/2
  Merge/1 -> TiSpan/1
  uSec per Sec/1 -> Product2/2
  Count per uSec/1 -> Divide1/2
  Data Store Read1/1 -> Product2/1
  Product2/1 -> Divide1/1
  Divide1/1 -> Subtract3/1, Divide2/1
  Max Counts/1 -> Product3/2, Divide2/2
  Divide2/1 -> Rounding/1
  Rounding/1 -> Product3/1
  Subtract3/1 -> Data Type Conversion2/1
  Product3/1 -> Subtract3/2
  If/1 -> NoWrapping/Action
  If/2 -> Wrapping/Action
  NoWrapping/1(Out1) -> Merge/1
  Wrapping/1(Out1) -> Merge/2

== system CF025A_GmFctDiArbn/GmFctDiArbn/GmFctDiArbnPer1/LoaSt_doesnt_equal_SwBasdMtgtn/CheckHwTqZeroAndHwAgZero/IfBothEotElpdTimeMet/OnCentrElpdTi/ElpdTi_Start/Copyright1 ==

== system CF025A_GmFctDiArbn/GmFctDiArbn/GmFctDiArbnPer1/LoaSt_doesnt_equal_SwBasdMtgtn/CheckHwTqZeroAndHwAgZero/IfBothEotElpdTimeMet/OnCentrElpdTi/ElpdTi_Start/GetRefTmr100MicroSec32bit ==
  note: 1 count = 100 uSec
  note: seconds
  note: microseconds
  note: counts
  note: Wrap-to-zero
  note: GetRefTmr100MicroSec32bit
  note: Created Aug 18, 2015
      | Modified Oct 21, 2015
      | Modified Oct 30, 2015
      | Kevin Derry
  CopyRight2 : Subsystem  Description=|  mask(Copyright Information){none=on}
      | Copyright info block.                                               
      |                                                                     
      | Place copyright information at the top of every subsystem in design.
      mask prompts: none "No parameters"
      mask help: Place copyright information at the top of every subsystem in design.
      mask Display:
      | NxtrConf = 'Nexteer Confidential';
      | 
      | sys = bdroot; %handle for the current model ("system")
      | first = get_param(sys,'Created');
      | if(isempty(first))
      |     first = datestr(now,'yyyy');
      | else
      |     first = first(end-3:end);  %year is last four digits
      | end
      | 
      | last = get_param(sys,'LastModifiedDate');
      | if isempty(last)
      |     last = datestr(now,'yyyy');
      | else
      |     last = last(end-3:end);
      | end
      | 
      | if strcmp(first,last)
      |     fprintf('%s -- Copyright %s Nexteer',NxtrConf,first)
      | else
      |     fprintf('%s -- %s%s- %s Nexteer',NxtrConf,char(169),first,last)
      | end
  Count per uSec : Constant  Value=0.01
  Data Store Read1 : DataStoreRead  DataStoreName=SimnTi
  Data Type Conversion1 : DataTypeConversion  OutDataTypeStr=uint32
  Divide1 : Product  Inputs=**
  Divide2 : Product  Inputs=*/
  Max Counts : Constant  Value=2^32-1
  Product1 : Product
  Product2 : Product
  Rounding : Rounding
  Subtract1 : Sum  Inputs=+-
  uSec per Sec : Constant  Value=1000000
  RefTmr : Outport
  wires:
  Product2/1 -> Subtract1/2
  Subtract1/1 -> Data Type Conversion1/1
  Rounding/1 -> Product2/1
  Divide2/1 -> Rounding/1
  Max Counts/1 -> Divide2/2, Product2/2
  Divide1/1 -> Divide2/1, Subtract1/1
  Product1/1 -> Divide1/1
  Count per uSec/1 -> Divide1/2
  uSec per Sec/1 -> Product1/2
  Data Type Conversion1/1 -> RefTmr/1
  Data Store Read1/1 -> Product1/1

== system CF025A_GmFctDiArbn/GmFctDiArbn/GmFctDiArbnPer1/LoaSt_doesnt_equal_SwBasdMtgtn/CheckHwTqZeroAndHwAgZero/IfBothEotElpdTimeMet/OnCentrElpdTi/ElpdTi_Zero/Copyright1 ==

== system CF025A_GmFctDiArbn/GmFctDiArbn/GmFctDiArbnPer1/LoaSt_doesnt_equal_SwBasdMtgtn/FcnDi_ElpdTi/ElpdTi_TiPassd/GetTiSpan100MicroSec32bit/NoWrapping/CopyRight2 ==

== system CF025A_GmFctDiArbn/GmFctDiArbn/GmFctDiArbnPer1/LoaSt_doesnt_equal_SwBasdMtgtn/FcnDi_ElpdTi/ElpdTi_TiPassd/GetTiSpan100MicroSec32bit/Wrapping/CopyRight2 ==

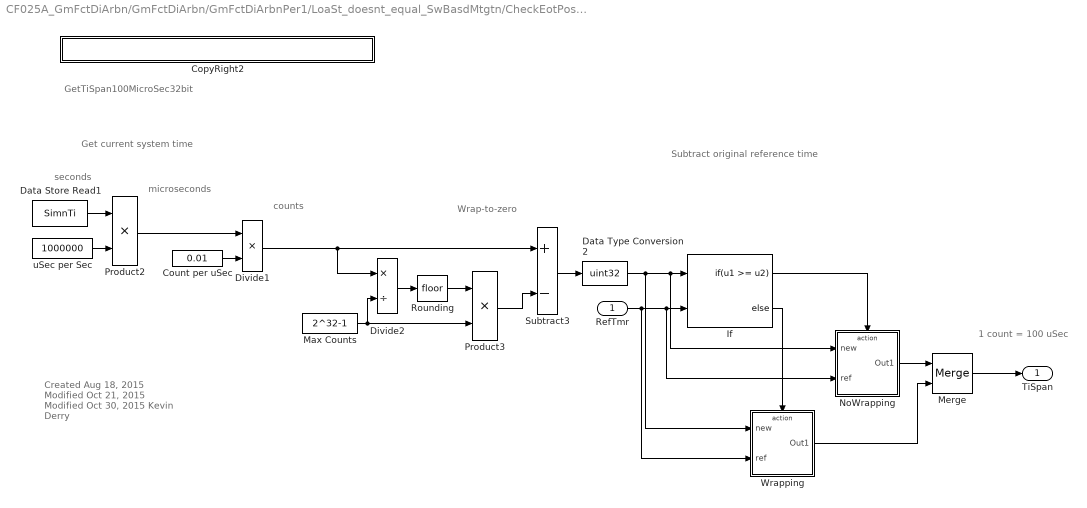
== system CF025A_GmFctDiArbn/GmFctDiArbn/GmFctDiArbnPer1/LoaSt_doesnt_equal_SwBasdMtgtn/CheckEotPosInRange/InProc/InRangeCcwDirection/InCcwEotElpdTi/ElpdTi_Check/GetTiSpan100MicroSec32bit ==
  note: Subtract original reference time
  note: seconds
  note: microseconds
  note: counts
  note: Wrap-to-zero
  note: 1 count = 100 uSec
  note: Get current system time
  note: GetTiSpan100MicroSec32bit
  note: Created Aug 18, 2015
      | Modified Oct 21, 2015
      | Modified Oct 30, 2015
      | Kevin Derry
  RefTmr : Inport
  CopyRight2 : Subsystem  Description=|  mask(Copyright Information){none=on}
      | Copyright info block.                                               
      |                                                                     
      | Place copyright information at the top of every subsystem in design.
      mask prompts: none "No parameters"
      mask help: Place copyright information at the top of every subsystem in design.
      mask Display:
      | NxtrConf = 'Nexteer Confidential';
      | 
      | sys = bdroot; %handle for the current model ("system")
      | first = get_param(sys,'Created');
      | if(isempty(first))
      |     first = datestr(now,'yyyy');
      | else
      |     first = first(end-3:end);  %year is last four digits
      | end
      | 
      | last = get_param(sys,'LastModifiedDate');
      | if isempty(last)
      |     last = datestr(now,'yyyy');
      | else
      |     last = last(end-3:end);
      | end
      | 
      | if strcmp(first,last)
      |     fprintf('%s -- Copyright %s Nexteer',NxtrConf,first)
      | else
      |     fprintf('%s -- %s%s- %s Nexteer',NxtrConf,char(169),first,last)
      | end
  Count per uSec : Constant  Value=0.01
  Data Store Read1 : DataStoreRead  DataStoreName=SimnTi
  Data Type Conversion2 : DataTypeConversion  OutDataTypeStr=uint32
  Divide1 : Product  Inputs=**
  Divide2 : Product  Inputs=*/
  If : If  NumInputs=2  IfExpression=u1 >= u2
  Max Counts : Constant  Value=2^32-1
  Merge : Merge
  NoWrapping : Subsystem  TreatAsAtomicUnit=on
  Product2 : Product
  Product3 : Product
  Rounding : Rounding
  Subtract3 : Sum  Inputs=+-
  Wrapping : Subsystem  TreatAsAtomicUnit=on
  uSec per Sec : Constant  Value=1000000
  TiSpan : Outport
  wires:
  Wrapping/1(Out1) -> Merge/2
  NoWrapping/1(Out1) -> Merge/1
  If/2 -> Wrapping/Action
  If/1 -> NoWrapping/Action
  Product3/1 -> Subtract3/2
  Subtract3/1 -> Data Type Conversion2/1
  Rounding/1 -> Product3/1
  Divide2/1 -> Rounding/1
  Max Counts/1 -> Divide2/2, Product3/2
  Divide1/1 -> Divide2/1, Subtract3/1
  Product2/1 -> Divide1/1
  Data Store Read1/1 -> Product2/1
  Count per uSec/1 -> Divide1/2
  uSec per Sec/1 -> Product2/2
  Merge/1 -> TiSpan/1
  RefTmr/1 -> If/2, NoWrapping/2(ref), Wrapping/2(ref)
  Data Type Conversion2/1 -> If/1, NoWrapping/1(new), Wrapping/1(new)

== system CF025A_GmFctDiArbn/GmFctDiArbn/GmFctDiArbnPer1/LoaSt_doesnt_equal_SwBasdMtgtn/CheckEotPosInRange/InProc/InRangeCcwDirection/InCcwEotElpdTi/ElpdTi_Start/GetRefTmr100MicroSec32bit ==
  note: Created Aug 18, 2015
      | Modified Oct 21, 2015
      | Modified Oct 30, 2015
      | Kevin Derry
  note: GetRefTmr100MicroSec32bit
  note: Wrap-to-zero
  note: counts
  note: microseconds
  note: seconds
  note: 1 count = 100 uSec
  CopyRight2 : Subsystem  Description=|  mask(Copyright Information){none=on}
      | Copyright info block.                                               
      |                                                                     
      | Place copyright information at the top of every subsystem in design.
      mask prompts: none "No parameters"
      mask help: Place copyright information at the top of every subsystem in design.
      mask Display:
      | NxtrConf = 'Nexteer Confidential';
      | 
      | sys = bdroot; %handle for the current model ("system")
      | first = get_param(sys,'Created');
      | if(isempty(first))
      |     first = datestr(now,'yyyy');
      | else
      |     first = first(end-3:end);  %year is last four digits
      | end
      | 
      | last = get_param(sys,'LastModifiedDate');
      | if isempty(last)
      |     last = datestr(now,'yyyy');
      | else
      |     last = last(end-3:end);
      | end
      | 
      | if strcmp(first,last)
      |     fprintf('%s -- Copyright %s Nexteer',NxtrConf,first)
      | else
      |     fprintf('%s -- %s%s- %s Nexteer',NxtrConf,char(169),first,last)
      | end
  Count per uSec : Constant  Value=0.01
  Data Store Read1 : DataStoreRead  DataStoreName=SimnTi
  Data Type Conversion1 : DataTypeConversion  OutDataTypeStr=uint32
  Divide1 : Product  Inputs=**
  Divide2 : Product  Inputs=*/
  Max Counts : Constant  Value=2^32-1
  Product1 : Product
  Product2 : Product
  Rounding : Rounding
  Subtract1 : Sum  Inputs=+-
  uSec per Sec : Constant  Value=1000000
  RefTmr : Outport
  wires:
  Data Store Read1/1 -> Product1/1
  Data Type Conversion1/1 -> RefTmr/1
  uSec per Sec/1 -> Product1/2
  Count per uSec/1 -> Divide1/2
  Product1/1 -> Divide1/1
  Divide1/1 -> Subtract1/1, Divide2/1
  Max Counts/1 -> Product2/2, Divide2/2
  Divide2/1 -> Rounding/1
  Rounding/1 -> Product2/1
  Subtract1/1 -> Data Type Conversion1/1
  Product2/1 -> Subtract1/2

== system CF025A_GmFctDiArbn/GmFctDiArbn/GmFctDiArbnPer1/LoaSt_doesnt_equal_SwBasdMtgtn/CheckEotPosInRange/InProc/InRangeCwDirection/InCwEotElpdTi/ElpdTi_Check/Copyright1 ==
